simulink model "VCU_CS75_12_30_test"  (R2014a)
settings: Solver=FixedStepDiscrete  StartTime=0.0  StopTime=25  FixedStep=0.0005  RelTol=1e-3
InitFcn:
  | PID_canshu
values from neighbouring files (symbols this model uses):
  D1 = ecucoder_cal(D1)    [PID_canshu.m]
  D2 = ecucoder_cal(D2)    [PID_canshu.m]
  D3 = ecucoder_cal(D3)    [PID_canshu.m]
  ErrorLimit = ecucoder_cal(ErrorLimit)    [PID_canshu.m]
  ErrorSumMax1 = ecucoder_cal(ErrorSumMax1)    [PID_canshu.m]
  ErrorSumMax2 = ecucoder_cal(ErrorSumMax2)    [PID_canshu.m]
  ErrorSumMax3 = ecucoder_cal(ErrorSumMax3)    [PID_canshu.m]
  I1 = ecucoder_cal(I1)    [PID_canshu.m]
  I2 = ecucoder_cal(I2)    [PID_canshu.m]
  I3 = ecucoder_cal(I3)    [PID_canshu.m]
  Limit1 = ecucoder_cal(Limit1)    [PID_canshu.m]
  Limit2 = ecucoder_cal(Limit2)    [PID_canshu.m]
  P1 = ecucoder_cal(P1)    [PID_canshu.m]
  P2 = ecucoder_cal(P2)    [PID_canshu.m]
  P3 = ecucoder_cal(P3)    [PID_canshu.m]
  T_buchang = ecucoder_cal(T_buchang)    [PID_canshu.m]
undefined symbols (not defined in the file or in its folder): ecucoder_acal, I_SW01_L, LaterlAngleCommand, LDW, RemoteAcclPosition
libraries: simulink x940, ec5744lib x41
(part 17 of 31)

== system VCU_CS75_12_30_test/长安CS75底盘程序，20ms一次/Output/CAN1_Tx/to2E5/ACC_2E5/ACC_AEBDecCtrlAvail ==
  ACC_AEBDecCtrlAvail : Inport
  ACC_AEBDecCtrlAvailRon : Rounding  Operator=round
  ACC_AEBDecCtrlAvail_1sat : Saturate  UpperLimit=128  LowerLimit=0
  ACC_AEBDecCtrlAvail_Convert : DataTypeConversion  OutDataTypeStr=uint8
  ACC_AEBDecCtrlAvail_Convert1 : DataTypeConversion  OutDataTypeStr=uint32
  ACC_AEBDecCtrlAvail_D : Product  Inputs=*/
  ACC_AEBDecCtrlAvail_F : Constant  OutDataTypeStr=single
  ACC_AEBDecCtrlAvail_L : simulink/Logic and Bit Operations/Bitwise Operator  logicop=AND  UseBitMask=on  BitMask=128  BitMaskRealWorld=Stored Integer
  ACC_AEBDecCtrlAvail_O : Constant  Value=0  OutDataTypeStr=single
  ACC_AEBDecCtrlAvail_S : ArithShift  BitShiftNumber=-7
  ACC_AEBDecCtrlAvail_sat : Saturate  UpperLimit=1  LowerLimit=0
  ACC_AEBDecCtrlAvail_st : Sum  Inputs=+-
  Constant{1..4,6..8} (7 alike) : Constant  Value=0  OutDataTypeStr=uint8
  output1 : Outport
  output2 : Outport  Port=2
  output3 : Outport  Port=3
  output4 : Outport  Port=4
  output5 : Outport  Port=5
  output6 : Outport  Port=6
  output7 : Outport  Port=7
  output8 : Outport  Port=8
  wires:
  ACC_AEBDecCtrlAvail/1 -> ACC_AEBDecCtrlAvail_sat/1
  ACC_AEBDecCtrlAvail_sat/1 -> ACC_AEBDecCtrlAvail_st/1
  ACC_AEBDecCtrlAvail_O/1 -> ACC_AEBDecCtrlAvail_st/2
  ACC_AEBDecCtrlAvail_st/1 -> ACC_AEBDecCtrlAvail_D/1
  ACC_AEBDecCtrlAvail_F/1 -> ACC_AEBDecCtrlAvail_D/2
  ACC_AEBDecCtrlAvail_D/1 -> ACC_AEBDecCtrlAvailRon/1
  ACC_AEBDecCtrlAvailRon/1 -> ACC_AEBDecCtrlAvail_S/1
  ACC_AEBDecCtrlAvail_S/1 -> ACC_AEBDecCtrlAvail_1sat/1
  ACC_AEBDecCtrlAvail_1sat/1 -> ACC_AEBDecCtrlAvail_Convert1/1
  ACC_AEBDecCtrlAvail_Convert1/1 -> ACC_AEBDecCtrlAvail_L/1
  ACC_AEBDecCtrlAvail_L/1 -> ACC_AEBDecCtrlAvail_Convert/1
  ACC_AEBDecCtrlAvail_Convert/1 -> output5/1
  Constant1/1 -> output1/1
  Constant2/1 -> output2/1
  Constant3/1 -> output3/1
  Constant4/1 -> output4/1
  Constant6/1 -> output6/1
  Constant7/1 -> output7/1
  Constant8/1 -> output8/1

== system VCU_CS75_12_30_test/长安CS75底盘程序，20ms一次/Output/CAN1_Tx/to2E5/ACC_2E5/ACC_AEBLVehilcehold ==
  ACC_AEBLVehilcehold : Inport
  ACC_AEBLVehilceholdRon : Rounding  Operator=round
  ACC_AEBLVehilcehold_1sat : Saturate  UpperLimit=4  LowerLimit=0
  ACC_AEBLVehilcehold_Convert : DataTypeConversion  OutDataTypeStr=uint8
  ACC_AEBLVehilcehold_Convert1 : DataTypeConversion  OutDataTypeStr=uint32
  ACC_AEBLVehilcehold_D : Product  Inputs=*/
  ACC_AEBLVehilcehold_F : Constant  OutDataTypeStr=single
  ACC_AEBLVehilcehold_L : simulink/Logic and Bit Operations/Bitwise Operator  logicop=AND  UseBitMask=on  BitMask=4  BitMaskRealWorld=Stored Integer
  ACC_AEBLVehilcehold_O : Constant  Value=0  OutDataTypeStr=single
  ACC_AEBLVehilcehold_S : ArithShift  BitShiftNumber=-2
  ACC_AEBLVehilcehold_sat : Saturate  UpperLimit=1  LowerLimit=0
  ACC_AEBLVehilcehold_st : Sum  Inputs=+-
  Constant{1..3,5..8} (7 alike) : Constant  Value=0  OutDataTypeStr=uint8
  output1 : Outport
  output2 : Outport  Port=2
  output3 : Outport  Port=3
  output4 : Outport  Port=4
  output5 : Outport  Port=5
  output6 : Outport  Port=6
  output7 : Outport  Port=7
  output8 : Outport  Port=8
  wires:
  ACC_AEBLVehilcehold/1 -> ACC_AEBLVehilcehold_sat/1
  ACC_AEBLVehilcehold_sat/1 -> ACC_AEBLVehilcehold_st/1
  ACC_AEBLVehilcehold_O/1 -> ACC_AEBLVehilcehold_st/2
  ACC_AEBLVehilcehold_st/1 -> ACC_AEBLVehilcehold_D/1
  ACC_AEBLVehilcehold_F/1 -> ACC_AEBLVehilcehold_D/2
  ACC_AEBLVehilcehold_D/1 -> ACC_AEBLVehilceholdRon/1
  ACC_AEBLVehilceholdRon/1 -> ACC_AEBLVehilcehold_S/1
  ACC_AEBLVehilcehold_S/1 -> ACC_AEBLVehilcehold_1sat/1
  ACC_AEBLVehilcehold_1sat/1 -> ACC_AEBLVehilcehold_Convert1/1
  ACC_AEBLVehilcehold_Convert1/1 -> ACC_AEBLVehilcehold_L/1
  ACC_AEBLVehilcehold_L/1 -> ACC_AEBLVehilcehold_Convert/1
  ACC_AEBLVehilcehold_Convert/1 -> output4/1
  Constant1/1 -> output1/1
  Constant2/1 -> output2/1
  Constant3/1 -> output3/1
  Constant5/1 -> output5/1
  Constant6/1 -> output6/1
  Constant7/1 -> output7/1
  Constant8/1 -> output8/1

== system VCU_CS75_12_30_test/长安CS75底盘程序，20ms一次/Output/CAN1_Tx/to2E5/ACC_2E5/ACC_AEBTargetDeceleration ==
  ACC_AEBTargetDeceleration : Inport
  ACC_AEBTargetDecelerationBitCov : DataTypeConversion  OutDataTypeStr=uint32
  ACC_AEBTargetDecelerationBitCov1 : DataTypeConversion  OutDataTypeStr=uint8
  ACC_AEBTargetDecelerationCOV : DataTypeConversion  OutDataTypeStr=uint8
  ACC_AEBTargetDecelerationCOV1 : DataTypeConversion  OutDataTypeStr=uint8
  ACC_AEBTargetDecelerationRon : Rounding  Operator=round
  ACC_AEBTargetDeceleration_1sat : Saturate  UpperLimit=2097120  LowerLimit=0
  ACC_AEBTargetDeceleration_And : simulink/Logic and Bit Operations/Bitwise Operator  logicop=AND  UseBitMask=off  NumInputPorts=2  BitMask=bin2dec('11011001')  BitMaskRealWorld=Stored Integer
  ACC_AEBTargetDeceleration_And1 : simulink/Logic and Bit Operations/Bitwise Operator  logicop=AND  UseBitMask=off  NumInputPorts=2  BitMask=bin2dec('11011001')  BitMaskRealWorld=Stored Integer
  ACC_AEBTargetDeceleration_And1_C : Constant  Value=255  OutDataTypeStr=uint32
  ACC_AEBTargetDeceleration_And_C : Constant  Value=65535
  ACC_AEBTargetDeceleration_Convert : DataTypeConversion  OutDataTypeStr=uint32
  ACC_AEBTargetDeceleration_D : Product  Inputs=*/
  ACC_AEBTargetDeceleration_D1 : Product  Inputs=*/
  ACC_AEBTargetDeceleration_D2 : Product  Inputs=*/
  ACC_AEBTargetDeceleration_F : Constant  Value=0.0005  OutDataTypeStr=single
  ACC_AEBTargetDeceleration_L : simulink/Logic and Bit Operations/Bitwise Operator  logicop=AND  UseBitMask=on  BitMask=2097120  BitMaskRealWorld=Stored Integer
  ACC_AEBTargetDeceleration_O : Constant  Value=-16  OutDataTypeStr=single
  ACC_AEBTargetDeceleration_S : ArithShift  BitShiftNumber=-5
  ACC_AEBTargetDeceleration_sat : Saturate  UpperLimit=16  LowerLimit=-16
  ACC_AEBTargetDeceleration_st : Sum  Inputs=+-
  ACC_AEBTargetDecelerationoutput1_C : Constant  Value=65536
  ACC_AEBTargetDecelerationoutput2_C : Constant  Value=256
  Constant{4..8} (5 alike) : Constant  Value=0  OutDataTypeStr=uint8
  output1 : Outport
  output2 : Outport  Port=2
  output3 : Outport  Port=3
  output4 : Outport  Port=4
  output5 : Outport  Port=5
  output6 : Outport  Port=6
  output7 : Outport  Port=7
  output8 : Outport  Port=8
  wires:
  ACC_AEBTargetDeceleration/1 -> ACC_AEBTargetDeceleration_sat/1
  ACC_AEBTargetDeceleration_sat/1 -> ACC_AEBTargetDeceleration_st/1
  ACC_AEBTargetDeceleration_O/1 -> ACC_AEBTargetDeceleration_st/2
  ACC_AEBTargetDeceleration_st/1 -> ACC_AEBTargetDeceleration_D/1
  ACC_AEBTargetDeceleration_F/1 -> ACC_AEBTargetDeceleration_D/2
  ACC_AEBTargetDeceleration_D/1 -> ACC_AEBTargetDecelerationRon/1
  ACC_AEBTargetDecelerationRon/1 -> ACC_AEBTargetDeceleration_S/1
  ACC_AEBTargetDeceleration_S/1 -> ACC_AEBTargetDeceleration_1sat/1
  ACC_AEBTargetDeceleration_1sat/1 -> ACC_AEBTargetDeceleration_Convert/1
  ACC_AEBTargetDeceleration_Convert/1 -> ACC_AEBTargetDeceleration_L/1
  ACC_AEBTargetDeceleration_L/1 -> ACC_AEBTargetDeceleration_D1/1, ACC_AEBTargetDeceleration_And/1, ACC_AEBTargetDeceleration_And1/1
  ACC_AEBTargetDecelerationoutput1_C/1 -> ACC_AEBTargetDeceleration_D1/2
  ACC_AEBTargetDeceleration_D1/1 -> ACC_AEBTargetDecelerationCOV/1
  ACC_AEBTargetDecelerationCOV/1 -> output1/1
  ACC_AEBTargetDeceleration_And_C/1 -> ACC_AEBTargetDecelerationBitCov/1
  ACC_AEBTargetDecelerationBitCov/1 -> ACC_AEBTargetDeceleration_And/2
  ACC_AEBTargetDeceleration_And/1 -> ACC_AEBTargetDeceleration_D2/1
  ACC_AEBTargetDecelerationoutput2_C/1 -> ACC_AEBTargetDeceleration_D2/2
  ACC_AEBTargetDeceleration_D2/1 -> ACC_AEBTargetDecelerationCOV1/1
  ACC_AEBTargetDecelerationCOV1/1 -> output2/1
  ACC_AEBTargetDeceleration_And1_C/1 -> ACC_AEBTargetDeceleration_And1/2
  ACC_AEBTargetDeceleration_And1/1 -> ACC_AEBTargetDecelerationBitCov1/1
  ACC_AEBTargetDecelerationBitCov1/1 -> output3/1
  Constant4/1 -> output4/1
  Constant5/1 -> output5/1
  Constant6/1 -> output6/1
  Constant7/1 -> output7/1
  Constant8/1 -> output8/1

== system VCU_CS75_12_30_test/长安CS75底盘程序，20ms一次/Output/CAN1_Tx/to2E5/ACC_2E5/ACC_AWBavailable ==
  ACC_AWBavailable : Inport
  ACC_AWBavailableRon : Rounding  Operator=round
  ACC_AWBavailable_1sat : Saturate  UpperLimit=128  LowerLimit=0
  ACC_AWBavailable_Convert : DataTypeConversion  OutDataTypeStr=uint8
  ACC_AWBavailable_Convert1 : DataTypeConversion  OutDataTypeStr=uint32
  ACC_AWBavailable_D : Product  Inputs=*/
  ACC_AWBavailable_F : Constant  OutDataTypeStr=single
  ACC_AWBavailable_L : simulink/Logic and Bit Operations/Bitwise Operator  logicop=AND  UseBitMask=on  BitMask=128  BitMaskRealWorld=Stored Integer
  ACC_AWBavailable_O : Constant  Value=0  OutDataTypeStr=single
  ACC_AWBavailable_S : ArithShift  BitShiftNumber=-7
  ACC_AWBavailable_sat : Saturate  UpperLimit=1  LowerLimit=0
  ACC_AWBavailable_st : Sum  Inputs=+-
  Constant{1..3,5..8} (7 alike) : Constant  Value=0  OutDataTypeStr=uint8
  output1 : Outport
  output2 : Outport  Port=2
  output3 : Outport  Port=3
  output4 : Outport  Port=4
  output5 : Outport  Port=5
  output6 : Outport  Port=6
  output7 : Outport  Port=7
  output8 : Outport  Port=8
  wires:
  ACC_AWBavailable/1 -> ACC_AWBavailable_sat/1
  ACC_AWBavailable_sat/1 -> ACC_AWBavailable_st/1
  ACC_AWBavailable_O/1 -> ACC_AWBavailable_st/2
  ACC_AWBavailable_st/1 -> ACC_AWBavailable_D/1
  ACC_AWBavailable_F/1 -> ACC_AWBavailable_D/2
  ACC_AWBavailable_D/1 -> ACC_AWBavailableRon/1
  ACC_AWBavailableRon/1 -> ACC_AWBavailable_S/1
  ACC_AWBavailable_S/1 -> ACC_AWBavailable_1sat/1
  ACC_AWBavailable_1sat/1 -> ACC_AWBavailable_Convert1/1
  ACC_AWBavailable_Convert1/1 -> ACC_AWBavailable_L/1
  ACC_AWBavailable_L/1 -> ACC_AWBavailable_Convert/1
  ACC_AWBavailable_Convert/1 -> output4/1
  Constant1/1 -> output1/1
  Constant2/1 -> output2/1
  Constant3/1 -> output3/1
  Constant5/1 -> output5/1
  Constant6/1 -> output6/1
  Constant7/1 -> output7/1
  Constant8/1 -> output8/1

== system VCU_CS75_12_30_test/长安CS75底盘程序，20ms一次/Output/CAN1_Tx/to2E5/ACC_2E5/ACC_AWBlevel ==
  ACC_AWBlevel : Inport
  ACC_AWBlevelRon : Rounding  Operator=round
  ACC_AWBlevel_1sat : Saturate  UpperLimit=15  LowerLimit=0
  ACC_AWBlevel_Convert : DataTypeConversion  OutDataTypeStr=uint8
  ACC_AWBlevel_Convert1 : DataTypeConversion  OutDataTypeStr=uint32
  ACC_AWBlevel_D : Product  Inputs=*/
  ACC_AWBlevel_F : Constant  OutDataTypeStr=single
  ACC_AWBlevel_L : simulink/Logic and Bit Operations/Bitwise Operator  logicop=AND  UseBitMask=on  BitMask=15  BitMaskRealWorld=Stored Integer
  ACC_AWBlevel_O : Constant  Value=0  OutDataTypeStr=single
  ACC_AWBlevel_S : ArithShift
  ACC_AWBlevel_sat : Saturate  UpperLimit=15  LowerLimit=0
  ACC_AWBlevel_st : Sum  Inputs=+-
  Constant{1..2,4..8} (7 alike) : Constant  Value=0  OutDataTypeStr=uint8
  output1 : Outport
  output2 : Outport  Port=2
  output3 : Outport  Port=3
  output4 : Outport  Port=4
  output5 : Outport  Port=5
  output6 : Outport  Port=6
  output7 : Outport  Port=7
  output8 : Outport  Port=8
  wires:
  ACC_AWBlevel/1 -> ACC_AWBlevel_sat/1
  ACC_AWBlevel_sat/1 -> ACC_AWBlevel_st/1
  ACC_AWBlevel_O/1 -> ACC_AWBlevel_st/2
  ACC_AWBlevel_st/1 -> ACC_AWBlevel_D/1
  ACC_AWBlevel_F/1 -> ACC_AWBlevel_D/2
  ACC_AWBlevel_D/1 -> ACC_AWBlevelRon/1
  ACC_AWBlevelRon/1 -> ACC_AWBlevel_S/1
  ACC_AWBlevel_S/1 -> ACC_AWBlevel_1sat/1
  ACC_AWBlevel_1sat/1 -> ACC_AWBlevel_Convert1/1
  ACC_AWBlevel_Convert1/1 -> ACC_AWBlevel_L/1
  ACC_AWBlevel_L/1 -> ACC_AWBlevel_Convert/1
  ACC_AWBlevel_Convert/1 -> output3/1
  Constant1/1 -> output1/1
  Constant2/1 -> output2/1
  Constant4/1 -> output4/1
  Constant5/1 -> output5/1
  Constant6/1 -> output6/1
  Constant7/1 -> output7/1
  Constant8/1 -> output8/1

== system VCU_CS75_12_30_test/长安CS75底盘程序，20ms一次/Output/CAN1_Tx/to2E5/ACC_2E5/ACC_AccTorqueReq ==
  ACC_AccTorqueReq : Inport
  ACC_AccTorqueReqBitCov : DataTypeConversion  OutDataTypeStr=uint8
  ACC_AccTorqueReqCOV : DataTypeConversion  OutDataTypeStr=uint8
  ACC_AccTorqueReqRon : Rounding  Operator=round
  ACC_AccTorqueReq_1sat : Saturate  UpperLimit=4092  LowerLimit=0
  ACC_AccTorqueReq_And : simulink/Logic and Bit Operations/Bitwise Operator  logicop=AND  UseBitMask=off  NumInputPorts=2  BitMask=bin2dec('11011001')  BitMaskRealWorld=Stored Integer
  ACC_AccTorqueReq_And_C : Constant  Value=255  OutDataTypeStr=uint32
  ACC_AccTorqueReq_Convert : DataTypeConversion  OutDataTypeStr=uint32
  ACC_AccTorqueReq_D : Product  Inputs=*/
  ACC_AccTorqueReq_D1 : Product  Inputs=*/
  ACC_AccTorqueReq_F : Constant  Value=0.09784  OutDataTypeStr=single
  ACC_AccTorqueReq_L : simulink/Logic and Bit Operations/Bitwise Operator  logicop=AND  UseBitMask=on  BitMask=4092  BitMaskRealWorld=Stored Integer
  ACC_AccTorqueReq_O : Constant  Value=0  OutDataTypeStr=single
  ACC_AccTorqueReq_S : ArithShift  BitShiftNumber=-2
  ACC_AccTorqueReq_sat : Saturate  UpperLimit=100.09032  LowerLimit=0
  ACC_AccTorqueReq_st : Sum  Inputs=+-
  ACC_AccTorqueReqoutput5_C : Constant  Value=256
  Constant{1..4,7..8} (6 alike) : Constant  Value=0  OutDataTypeStr=uint8
  output1 : Outport
  output2 : Outport  Port=2
  output3 : Outport  Port=3
  output4 : Outport  Port=4
  output5 : Outport  Port=5
  output6 : Outport  Port=6
  output7 : Outport  Port=7
  output8 : Outport  Port=8
  wires:
  ACC_AccTorqueReq/1 -> ACC_AccTorqueReq_sat/1
  ACC_AccTorqueReq_sat/1 -> ACC_AccTorqueReq_st/1
  ACC_AccTorqueReq_O/1 -> ACC_AccTorqueReq_st/2
  ACC_AccTorqueReq_st/1 -> ACC_AccTorqueReq_D/1
  ACC_AccTorqueReq_F/1 -> ACC_AccTorqueReq_D/2
  ACC_AccTorqueReq_D/1 -> ACC_AccTorqueReqRon/1
  ACC_AccTorqueReqRon/1 -> ACC_AccTorqueReq_S/1
  ACC_AccTorqueReq_S/1 -> ACC_AccTorqueReq_1sat/1
  ACC_AccTorqueReq_1sat/1 -> ACC_AccTorqueReq_Convert/1
  ACC_AccTorqueReq_Convert/1 -> ACC_AccTorqueReq_L/1
  ACC_AccTorqueReq_L/1 -> ACC_AccTorqueReq_D1/1, ACC_AccTorqueReq_And/1
  ACC_AccTorqueReqoutput5_C/1 -> ACC_AccTorqueReq_D1/2
  ACC_AccTorqueReq_D1/1 -> ACC_AccTorqueReqCOV/1
  ACC_AccTorqueReqCOV/1 -> output5/1
  ACC_AccTorqueReq_And_C/1 -> ACC_AccTorqueReq_And/2
  ACC_AccTorqueReq_And/1 -> ACC_AccTorqueReqBitCov/1
  ACC_AccTorqueReqBitCov/1 -> output6/1
  Constant1/1 -> output1/1
  Constant2/1 -> output2/1
  Constant3/1 -> output3/1
  Constant4/1 -> output4/1
  Constant7/1 -> output7/1
  Constant8/1 -> output8/1

== system VCU_CS75_12_30_test/长安CS75底盘程序，20ms一次/Output/CAN1_Tx/to2E5/ACC_2E5/ACC_AccTrqReqEnable ==
  ACC_AccTrqReqEnable : Inport
  ACC_AccTrqReqEnableRon : Rounding  Operator=round
  ACC_AccTrqReqEnable_1sat : Saturate  UpperLimit=128  LowerLimit=0
  ACC_AccTrqReqEnable_Convert : DataTypeConversion  OutDataTypeStr=uint8
  ACC_AccTrqReqEnable_Convert1 : DataTypeConversion  OutDataTypeStr=uint32
  ACC_AccTrqReqEnable_D : Product  Inputs=*/
  ACC_AccTrqReqEnable_F : Constant  OutDataTypeStr=single
  ACC_AccTrqReqEnable_L : simulink/Logic and Bit Operations/Bitwise Operator  logicop=AND  UseBitMask=on  BitMask=128  BitMaskRealWorld=Stored Integer
  ACC_AccTrqReqEnable_O : Constant  Value=0  OutDataTypeStr=single
  ACC_AccTrqReqEnable_S : ArithShift  BitShiftNumber=-7
  ACC_AccTrqReqEnable_sat : Saturate  UpperLimit=1  LowerLimit=0
  ACC_AccTrqReqEnable_st : Sum  Inputs=+-
  Constant{2..8} (7 alike) : Constant  Value=0  OutDataTypeStr=uint8
  output1 : Outport
  output2 : Outport  Port=2
  output3 : Outport  Port=3
  output4 : Outport  Port=4
  output5 : Outport  Port=5
  output6 : Outport  Port=6
  output7 : Outport  Port=7
  output8 : Outport  Port=8
  wires:
  ACC_AccTrqReqEnable/1 -> ACC_AccTrqReqEnable_sat/1
  ACC_AccTrqReqEnable_sat/1 -> ACC_AccTrqReqEnable_st/1
  ACC_AccTrqReqEnable_O/1 -> ACC_AccTrqReqEnable_st/2
  ACC_AccTrqReqEnable_st/1 -> ACC_AccTrqReqEnable_D/1
  ACC_AccTrqReqEnable_F/1 -> ACC_AccTrqReqEnable_D/2
  ACC_AccTrqReqEnable_D/1 -> ACC_AccTrqReqEnableRon/1
  ACC_AccTrqReqEnableRon/1 -> ACC_AccTrqReqEnable_S/1
  ACC_AccTrqReqEnable_S/1 -> ACC_AccTrqReqEnable_1sat/1
  ACC_AccTrqReqEnable_1sat/1 -> ACC_AccTrqReqEnable_Convert1/1
  ACC_AccTrqReqEnable_Convert1/1 -> ACC_AccTrqReqEnable_L/1
  ACC_AccTrqReqEnable_L/1 -> ACC_AccTrqReqEnable_Convert/1
  ACC_AccTrqReqEnable_Convert/1 -> output1/1
  Constant2/1 -> output2/1
  Constant3/1 -> output3/1
  Constant4/1 -> output4/1
  Constant5/1 -> output5/1
  Constant6/1 -> output6/1
  Constant7/1 -> output7/1
  Constant8/1 -> output8/1

== system VCU_CS75_12_30_test/长安CS75底盘程序，20ms一次/Output/CAN1_Tx/to2E5/ACC_2E5/ACC_CheckSum ==
  ACC_CheckSum : Inport
  ACC_CheckSumRon : Rounding  Operator=round
  ACC_CheckSum_1sat : Saturate  UpperLimit=255  LowerLimit=0
  ACC_CheckSum_Convert : DataTypeConversion  OutDataTypeStr=uint8
  ACC_CheckSum_Convert1 : DataTypeConversion  OutDataTypeStr=uint32
  ACC_CheckSum_D : Product  Inputs=*/
  ACC_CheckSum_F : Constant  OutDataTypeStr=single
  ACC_CheckSum_L : simulink/Logic and Bit Operations/Bitwise Operator  logicop=AND  UseBitMask=on  BitMask=255  BitMaskRealWorld=Stored Integer
  ACC_CheckSum_O : Constant  Value=0  OutDataTypeStr=single
  ACC_CheckSum_S : ArithShift
  ACC_CheckSum_sat : Saturate  UpperLimit=255  LowerLimit=0
  ACC_CheckSum_st : Sum  Inputs=+-
  Constant{1..7} (7 alike) : Constant  Value=0  OutDataTypeStr=uint8
  output1 : Outport
  output2 : Outport  Port=2
  output3 : Outport  Port=3
  output4 : Outport  Port=4
  output5 : Outport  Port=5
  output6 : Outport  Port=6
  output7 : Outport  Port=7
  output8 : Outport  Port=8
  wires:
  ACC_CheckSum/1 -> ACC_CheckSum_sat/1
  ACC_CheckSum_sat/1 -> ACC_CheckSum_st/1
  ACC_CheckSum_O/1 -> ACC_CheckSum_st/2
  ACC_CheckSum_st/1 -> ACC_CheckSum_D/1
  ACC_CheckSum_F/1 -> ACC_CheckSum_D/2
  ACC_CheckSum_D/1 -> ACC_CheckSumRon/1
  ACC_CheckSumRon/1 -> ACC_CheckSum_S/1
  ACC_CheckSum_S/1 -> ACC_CheckSum_1sat/1
  ACC_CheckSum_1sat/1 -> ACC_CheckSum_Convert1/1
  ACC_CheckSum_Convert1/1 -> ACC_CheckSum_L/1
  ACC_CheckSum_L/1 -> ACC_CheckSum_Convert/1
  ACC_CheckSum_Convert/1 -> output8/1
  Constant1/1 -> output1/1
  Constant2/1 -> output2/1
  Constant3/1 -> output3/1
  Constant4/1 -> output4/1
  Constant5/1 -> output5/1
  Constant6/1 -> output6/1
  Constant7/1 -> output7/1

== system VCU_CS75_12_30_test/长安CS75底盘程序，20ms一次/Output/CAN1_Tx/to2E5/ACC_2E5/ACC_ESPPrefill ==
  ACC_ESPPrefill : Inport
  ACC_ESPPrefillRon : Rounding  Operator=round
  ACC_ESPPrefill_1sat : Saturate  UpperLimit=64  LowerLimit=0
  ACC_ESPPrefill_Convert : DataTypeConversion  OutDataTypeStr=uint8
  ACC_ESPPrefill_Convert1 : DataTypeConversion  OutDataTypeStr=uint32
  ACC_ESPPrefill_D : Product  Inputs=*/
  ACC_ESPPrefill_F : Constant  OutDataTypeStr=single
  ACC_ESPPrefill_L : simulink/Logic and Bit Operations/Bitwise Operator  logicop=AND  UseBitMask=on  BitMask=64  BitMaskRealWorld=Stored Integer
  ACC_ESPPrefill_O : Constant  Value=0  OutDataTypeStr=single
  ACC_ESPPrefill_S : ArithShift  BitShiftNumber=-6
  ACC_ESPPrefill_sat : Saturate  UpperLimit=1  LowerLimit=0
  ACC_ESPPrefill_st : Sum  Inputs=+-
  Constant{1..3,5..8} (7 alike) : Constant  Value=0  OutDataTypeStr=uint8
  output1 : Outport
  output2 : Outport  Port=2
  output3 : Outport  Port=3
  output4 : Outport  Port=4
  output5 : Outport  Port=5
  output6 : Outport  Port=6
  output7 : Outport  Port=7
  output8 : Outport  Port=8
  wires:
  ACC_ESPPrefill/1 -> ACC_ESPPrefill_sat/1
  ACC_ESPPrefill_sat/1 -> ACC_ESPPrefill_st/1
  ACC_ESPPrefill_O/1 -> ACC_ESPPrefill_st/2
  ACC_ESPPrefill_st/1 -> ACC_ESPPrefill_D/1
  ACC_ESPPrefill_F/1 -> ACC_ESPPrefill_D/2
  ACC_ESPPrefill_D/1 -> ACC_ESPPrefillRon/1
  ACC_ESPPrefillRon/1 -> ACC_ESPPrefill_S/1
  ACC_ESPPrefill_S/1 -> ACC_ESPPrefill_1sat/1
  ACC_ESPPrefill_1sat/1 -> ACC_ESPPrefill_Convert1/1
  ACC_ESPPrefill_Convert1/1 -> ACC_ESPPrefill_L/1
  ACC_ESPPrefill_L/1 -> ACC_ESPPrefill_Convert/1
  ACC_ESPPrefill_Convert/1 -> output4/1
  Constant1/1 -> output1/1
  Constant2/1 -> output2/1
  Constant3/1 -> output3/1
  Constant5/1 -> output5/1
  Constant6/1 -> output6/1
  Constant7/1 -> output7/1
  Constant8/1 -> output8/1

== system VCU_CS75_12_30_test/长安CS75底盘程序，20ms一次/Output/CAN1_Tx/to2E5/ACC_2E5/ACC_PCWPenable ==
  ACC_PCWPenable : Inport
  ACC_PCWPenableRon : Rounding  Operator=round
  ACC_PCWPenable_1sat : Saturate  UpperLimit=32  LowerLimit=0
  ACC_PCWPenable_Convert : DataTypeConversion  OutDataTypeStr=uint8
  ACC_PCWPenable_Convert1 : DataTypeConversion  OutDataTypeStr=uint32
  ACC_PCWPenable_D : Product  Inputs=*/
  ACC_PCWPenable_F : Constant  OutDataTypeStr=single
  ACC_PCWPenable_L : simulink/Logic and Bit Operations/Bitwise Operator  logicop=AND  UseBitMask=on  BitMask=32  BitMaskRealWorld=Stored Integer
  ACC_PCWPenable_O : Constant  Value=0  OutDataTypeStr=single
  ACC_PCWPenable_S : ArithShift  BitShiftNumber=-5
  ACC_PCWPenable_sat : Saturate  UpperLimit=1  LowerLimit=0
  ACC_PCWPenable_st : Sum  Inputs=+-
  Constant{1..3,5..8} (7 alike) : Constant  Value=0  OutDataTypeStr=uint8
  output1 : Outport
  output2 : Outport  Port=2
  output3 : Outport  Port=3
  output4 : Outport  Port=4
  output5 : Outport  Port=5
  output6 : Outport  Port=6
  output7 : Outport  Port=7
  output8 : Outport  Port=8
  wires:
  ACC_PCWPenable/1 -> ACC_PCWPenable_sat/1
  ACC_PCWPenable_sat/1 -> ACC_PCWPenable_st/1
  ACC_PCWPenable_O/1 -> ACC_PCWPenable_st/2
  ACC_PCWPenable_st/1 -> ACC_PCWPenable_D/1
  ACC_PCWPenable_F/1 -> ACC_PCWPenable_D/2
  ACC_PCWPenable_D/1 -> ACC_PCWPenableRon/1
  ACC_PCWPenableRon/1 -> ACC_PCWPenable_S/1
  ACC_PCWPenable_S/1 -> ACC_PCWPenable_1sat/1
  ACC_PCWPenable_1sat/1 -> ACC_PCWPenable_Convert1/1
  ACC_PCWPenable_Convert1/1 -> ACC_PCWPenable_L/1
  ACC_PCWPenable_L/1 -> ACC_PCWPenable_Convert/1
  ACC_PCWPenable_Convert/1 -> output4/1
  Constant1/1 -> output1/1
  Constant2/1 -> output2/1
  Constant3/1 -> output3/1
  Constant5/1 -> output5/1
  Constant6/1 -> output6/1
  Constant7/1 -> output7/1
  Constant8/1 -> output8/1

== system VCU_CS75_12_30_test/长安CS75底盘程序，20ms一次/Output/CAN1_Tx/to2E5/ACC_2E5/ACC_PCWPreWarning ==
  ACC_PCWPreWarning : Inport
  ACC_PCWPreWarningRon : Rounding  Operator=round
  ACC_PCWPreWarning_1sat : Saturate  UpperLimit=8  LowerLimit=0
  ACC_PCWPreWarning_Convert : DataTypeConversion  OutDataTypeStr=uint8
  ACC_PCWPreWarning_Convert1 : DataTypeConversion  OutDataTypeStr=uint32
  ACC_PCWPreWarning_D : Product  Inputs=*/
  ACC_PCWPreWarning_F : Constant  OutDataTypeStr=single
  ACC_PCWPreWarning_L : simulink/Logic and Bit Operations/Bitwise Operator  logicop=AND  UseBitMask=on  BitMask=8  BitMaskRealWorld=Stored Integer
  ACC_PCWPreWarning_O : Constant  Value=0  OutDataTypeStr=single
  ACC_PCWPreWarning_S : ArithShift  BitShiftNumber=-3
  ACC_PCWPreWarning_sat : Saturate  UpperLimit=0  LowerLimit=0
  ACC_PCWPreWarning_st : Sum  Inputs=+-
  Constant{1..3,5..8} (7 alike) : Constant  Value=0  OutDataTypeStr=uint8
  output1 : Outport
  output2 : Outport  Port=2
  output3 : Outport  Port=3
  output4 : Outport  Port=4
  output5 : Outport  Port=5
  output6 : Outport  Port=6
  output7 : Outport  Port=7
  output8 : Outport  Port=8
  wires:
  ACC_PCWPreWarning/1 -> ACC_PCWPreWarning_sat/1
  ACC_PCWPreWarning_sat/1 -> ACC_PCWPreWarning_st/1
  ACC_PCWPreWarning_O/1 -> ACC_PCWPreWarning_st/2
  ACC_PCWPreWarning_st/1 -> ACC_PCWPreWarning_D/1
  ACC_PCWPreWarning_F/1 -> ACC_PCWPreWarning_D/2
  ACC_PCWPreWarning_D/1 -> ACC_PCWPreWarningRon/1
  ACC_PCWPreWarningRon/1 -> ACC_PCWPreWarning_S/1
  ACC_PCWPreWarning_S/1 -> ACC_PCWPreWarning_1sat/1
  ACC_PCWPreWarning_1sat/1 -> ACC_PCWPreWarning_Convert1/1
  ACC_PCWPreWarning_Convert1/1 -> ACC_PCWPreWarning_L/1
  ACC_PCWPreWarning_L/1 -> ACC_PCWPreWarning_Convert/1
  ACC_PCWPreWarning_Convert/1 -> output4/1
  Constant1/1 -> output1/1
  Constant2/1 -> output2/1
  Constant3/1 -> output3/1
  Constant5/1 -> output5/1
  Constant6/1 -> output6/1
  Constant7/1 -> output7/1
  Constant8/1 -> output8/1

== system VCU_CS75_12_30_test/长安CS75底盘程序，20ms一次/Output/CAN1_Tx/to2E5/ACC_2E5/ACC_PCW_LatentWarning ==
  ACC_PCW_LatentWarning : Inport
  ACC_PCW_LatentWarningRon : Rounding  Operator=round
  ACC_PCW_LatentWarning_1sat : Saturate  UpperLimit=16  LowerLimit=0
  ACC_PCW_LatentWarning_Convert : DataTypeConversion  OutDataTypeStr=uint8
  ACC_PCW_LatentWarning_Convert1 : DataTypeConversion  OutDataTypeStr=uint32
  ACC_PCW_LatentWarning_D : Product  Inputs=*/
  ACC_PCW_LatentWarning_F : Constant  OutDataTypeStr=single
  ACC_PCW_LatentWarning_L : simulink/Logic and Bit Operations/Bitwise Operator  logicop=AND  UseBitMask=on  BitMask=16  BitMaskRealWorld=Stored Integer
  ACC_PCW_LatentWarning_O : Constant  Value=0  OutDataTypeStr=single
  ACC_PCW_LatentWarning_S : ArithShift  BitShiftNumber=-4
  ACC_PCW_LatentWarning_sat : Saturate  UpperLimit=0  LowerLimit=0
  ACC_PCW_LatentWarning_st : Sum  Inputs=+-
  Constant{1..3,5..8} (7 alike) : Constant  Value=0  OutDataTypeStr=uint8
  output1 : Outport
  output2 : Outport  Port=2
  output3 : Outport  Port=3
  output4 : Outport  Port=4
  output5 : Outport  Port=5
  output6 : Outport  Port=6
  output7 : Outport  Port=7
  output8 : Outport  Port=8
  wires:
  ACC_PCW_LatentWarning/1 -> ACC_PCW_LatentWarning_sat/1
  ACC_PCW_LatentWarning_sat/1 -> ACC_PCW_LatentWarning_st/1
  ACC_PCW_LatentWarning_O/1 -> ACC_PCW_LatentWarning_st/2
  ACC_PCW_LatentWarning_st/1 -> ACC_PCW_LatentWarning_D/1
  ACC_PCW_LatentWarning_F/1 -> ACC_PCW_LatentWarning_D/2
  ACC_PCW_LatentWarning_D/1 -> ACC_PCW_LatentWarningRon/1
  ACC_PCW_LatentWarningRon/1 -> ACC_PCW_LatentWarning_S/1
  ACC_PCW_LatentWarning_S/1 -> ACC_PCW_LatentWarning_1sat/1
  ACC_PCW_LatentWarning_1sat/1 -> ACC_PCW_LatentWarning_Convert1/1
  ACC_PCW_LatentWarning_Convert1/1 -> ACC_PCW_LatentWarning_L/1
  ACC_PCW_LatentWarning_L/1 -> ACC_PCW_LatentWarning_Convert/1
  ACC_PCW_LatentWarning_Convert/1 -> output4/1
  Constant1/1 -> output1/1
  Constant2/1 -> output2/1
  Constant3/1 -> output3/1
  Constant5/1 -> output5/1
  Constant6/1 -> output6/1
  Constant7/1 -> output7/1
  Constant8/1 -> output8/1

== system VCU_CS75_12_30_test/长安CS75底盘程序，20ms一次/Output/CAN1_Tx/to2E5/ACC_2E5/ACC_RollingCounter ==
  ACC_RollingCounter : Inport
  ACC_RollingCounterRon : Rounding  Operator=round
  ACC_RollingCounter_1sat : Saturate  UpperLimit=15  LowerLimit=0
  ACC_RollingCounter_Convert : DataTypeConversion  OutDataTypeStr=uint8
  ACC_RollingCounter_Convert1 : DataTypeConversion  OutDataTypeStr=uint32
  ACC_RollingCounter_D : Product  Inputs=*/
  ACC_RollingCounter_F : Constant  OutDataTypeStr=single
  ACC_RollingCounter_L : simulink/Logic and Bit Operations/Bitwise Operator  logicop=AND  UseBitMask=on  BitMask=15  BitMaskRealWorld=Stored Integer
  ACC_RollingCounter_O : Constant  Value=0  OutDataTypeStr=single
  ACC_RollingCounter_S : ArithShift
  ACC_RollingCounter_sat : Saturate  UpperLimit=15  LowerLimit=0
  ACC_RollingCounter_st : Sum  Inputs=+-
  Constant{1..6,8} (7 alike) : Constant  Value=0  OutDataTypeStr=uint8
  output1 : Outport
  output2 : Outport  Port=2
  output3 : Outport  Port=3
  output4 : Outport  Port=4
  output5 : Outport  Port=5
  output6 : Outport  Port=6
  output7 : Outport  Port=7
  output8 : Outport  Port=8
  wires:
  ACC_RollingCounter/1 -> ACC_RollingCounter_sat/1
  ACC_RollingCounter_sat/1 -> ACC_RollingCounter_st/1
  ACC_RollingCounter_O/1 -> ACC_RollingCounter_st/2
  ACC_RollingCounter_st/1 -> ACC_RollingCounter_D/1
  ACC_RollingCounter_F/1 -> ACC_RollingCounter_D/2
  ACC_RollingCounter_D/1 -> ACC_RollingCounterRon/1
  ACC_RollingCounterRon/1 -> ACC_RollingCounter_S/1
  ACC_RollingCounter_S/1 -> ACC_RollingCounter_1sat/1
  ACC_RollingCounter_1sat/1 -> ACC_RollingCounter_Convert1/1
  ACC_RollingCounter_Convert1/1 -> ACC_RollingCounter_L/1
  ACC_RollingCounter_L/1 -> ACC_RollingCounter_Convert/1
  ACC_RollingCounter_Convert/1 -> output7/1
  Constant1/1 -> output1/1
  Constant2/1 -> output2/1
  Constant3/1 -> output3/1
  Constant4/1 -> output4/1
  Constant5/1 -> output5/1
  Constant6/1 -> output6/1
  Constant8/1 -> output8/1

== system VCU_CS75_12_30_test/长安CS75底盘程序，20ms一次/Output/CAN1_Tx/to2E5/ACC_2E5/ACC_TextInfoForDriver ==
  ACC_TextInfoForDriver : Inport
  ACC_TextInfoForDriverBitCov : DataTypeConversion  OutDataTypeStr=uint8
  ACC_TextInfoForDriverCOV : DataTypeConversion  OutDataTypeStr=uint8
  ACC_TextInfoForDriverRon : Rounding  Operator=round
  ACC_TextInfoForDriver_1sat : Saturate  UpperLimit=992  LowerLimit=0
  ACC_TextInfoForDriver_And : simulink/Logic and Bit Operations/Bitwise Operator  logicop=AND  UseBitMask=off  NumInputPorts=2  BitMask=bin2dec('11011001')  BitMaskRealWorld=Stored Integer
  ACC_TextInfoForDriver_And_C : Constant  Value=255  OutDataTypeStr=uint32
  ACC_TextInfoForDriver_Convert : DataTypeConversion  OutDataTypeStr=uint32
  ACC_TextInfoForDriver_D : Product  Inputs=*/
  ACC_TextInfoForDriver_D1 : Product  Inputs=*/
  ACC_TextInfoForDriver_F : Constant  OutDataTypeStr=single
  ACC_TextInfoForDriver_L : simulink/Logic and Bit Operations/Bitwise Operator  logicop=AND  UseBitMask=on  BitMask=992  BitMaskRealWorld=Stored Integer
  ACC_TextInfoForDriver_O : Constant  Value=0  OutDataTypeStr=single
  ACC_TextInfoForDriver_S : ArithShift  BitShiftNumber=-5
  ACC_TextInfoForDriver_sat : Saturate  UpperLimit=31  LowerLimit=0
  ACC_TextInfoForDriver_st : Sum  Inputs=+-
  ACC_TextInfoForDriveroutput6_C : Constant  Value=256
  Constant{1..5,8} (6 alike) : Constant  Value=0  OutDataTypeStr=uint8
  output1 : Outport
  output2 : Outport  Port=2
  output3 : Outport  Port=3
  output4 : Outport  Port=4
  output5 : Outport  Port=5
  output6 : Outport  Port=6
  output7 : Outport  Port=7
  output8 : Outport  Port=8
  wires:
  ACC_TextInfoForDriver/1 -> ACC_TextInfoForDriver_sat/1
  ACC_TextInfoForDriver_sat/1 -> ACC_TextInfoForDriver_st/1
  ACC_TextInfoForDriver_O/1 -> ACC_TextInfoForDriver_st/2
  ACC_TextInfoForDriver_st/1 -> ACC_TextInfoForDriver_D/1
  ACC_TextInfoForDriver_F/1 -> ACC_TextInfoForDriver_D/2
  ACC_TextInfoForDriver_D/1 -> ACC_TextInfoForDriverRon/1
  ACC_TextInfoForDriverRon/1 -> ACC_TextInfoForDriver_S/1
  ACC_TextInfoForDriver_S/1 -> ACC_TextInfoForDriver_1sat/1
  ACC_TextInfoForDriver_1sat/1 -> ACC_TextInfoForDriver_Convert/1
  ACC_TextInfoForDriver_Convert/1 -> ACC_TextInfoForDriver_L/1
  ACC_TextInfoForDriver_L/1 -> ACC_TextInfoForDriver_D1/1, ACC_TextInfoForDriver_And/1
  ACC_TextInfoForDriveroutput6_C/1 -> ACC_TextInfoForDriver_D1/2
  ACC_TextInfoForDriver_D1/1 -> ACC_TextInfoForDriverCOV/1
  ACC_TextInfoForDriverCOV/1 -> output6/1
  ACC_TextInfoForDriver_And_C/1 -> ACC_TextInfoForDriver_And/2
  ACC_TextInfoForDriver_And/1 -> ACC_TextInfoForDriverBitCov/1
  ACC_TextInfoForDriverBitCov/1 -> output7/1
  Constant1/1 -> output1/1
  Constant2/1 -> output2/1
  Constant3/1 -> output3/1
  Constant4/1 -> output4/1
  Constant5/1 -> output5/1
  Constant8/1 -> output8/1

== system VCU_CS75_12_30_test/长安CS75底盘程序，20ms一次/Output/Subsystem/28A/APA_28A/APA_CheckSum ==
  APA_CheckSum : Inport
  APA_CheckSumRon : Rounding  Operator=round
  APA_CheckSum_1sat : Saturate  UpperLimit=255  LowerLimit=0
  APA_CheckSum_Convert : DataTypeConversion  OutDataTypeStr=uint8
  APA_CheckSum_Convert1 : DataTypeConversion  OutDataTypeStr=uint32
  APA_CheckSum_D : Product  Inputs=*/
  APA_CheckSum_F : Constant  OutDataTypeStr=single
  APA_CheckSum_L : simulink/Logic and Bit Operations/Bitwise Operator  logicop=AND  UseBitMask=on  BitMask=255  BitMaskRealWorld=Stored Integer
  APA_CheckSum_O : Constant  Value=0  OutDataTypeStr=single
  APA_CheckSum_S : ArithShift
  APA_CheckSum_sat : Saturate  UpperLimit=255  LowerLimit=0
  APA_CheckSum_st : Sum  Inputs=+-
  Constant{1..7} (7 alike) : Constant  Value=0  OutDataTypeStr=uint8
  output1 : Outport
  output2 : Outport  Port=2
  output3 : Outport  Port=3
  output4 : Outport  Port=4
  output5 : Outport  Port=5
  output6 : Outport  Port=6
  output7 : Outport  Port=7
  output8 : Outport  Port=8
  wires:
  Constant7/1 -> output7/1
  Constant6/1 -> output6/1
  Constant5/1 -> output5/1
  Constant4/1 -> output4/1
  Constant3/1 -> output3/1
  Constant2/1 -> output2/1
  Constant1/1 -> output1/1
  APA_CheckSum_Convert/1 -> output8/1
  APA_CheckSum_L/1 -> APA_CheckSum_Convert/1
  APA_CheckSum_Convert1/1 -> APA_CheckSum_L/1
  APA_CheckSum_1sat/1 -> APA_CheckSum_Convert1/1
  APA_CheckSum_S/1 -> APA_CheckSum_1sat/1
  APA_CheckSumRon/1 -> APA_CheckSum_S/1
  APA_CheckSum_D/1 -> APA_CheckSumRon/1
  APA_CheckSum_F/1 -> APA_CheckSum_D/2
  APA_CheckSum_st/1 -> APA_CheckSum_D/1
  APA_CheckSum_O/1 -> APA_CheckSum_st/2
  APA_CheckSum_sat/1 -> APA_CheckSum_st/1
  APA_CheckSum/1 -> APA_CheckSum_sat/1

== system VCU_CS75_12_30_test/长安CS75底盘程序，20ms一次/Output/Subsystem/28A/APA_28A/APA_EPSAngleReq ==
  APA_EPSAngleReq : Inport
  APA_EPSAngleReqABS : Abs
  APA_EPSAngleReqBitCov : DataTypeConversion  OutDataTypeStr=uint32
  APA_EPSAngleReqBitCov1 : DataTypeConversion  OutDataTypeStr=uint8
  APA_EPSAngleReqCOV : DataTypeConversion  OutDataTypeStr=uint8
  APA_EPSAngleReqCOV1 : DataTypeConversion  OutDataTypeStr=uint8
  APA_EPSAngleReqCS : ArithShift  BitShiftNumber=-16
  APA_EPSAngleReqConS : Constant  OutDataTypeStr=single
  APA_EPSAngleReqCosR : Constant  Value=0  OutDataTypeStr=uint8
  APA_EPSAngleReqROP : RelationalOperator  Operator=<  OutDataTypeStr=boolean
  APA_EPSAngleReqRon : Rounding  Operator=round
  APA_EPSAngleReqSW : Switch  Criteria=u2 ~= 0
  APA_EPSAngleReq_1sat : Saturate  UpperLimit=1048560  LowerLimit=0
  APA_EPSAngleReq_And : simulink/Logic and Bit Operations/Bitwise Operator  logicop=AND  UseBitMask=off  NumInputPorts=2  BitMask=bin2dec('11011001')  BitMaskRealWorld=Stored Integer
  APA_EPSAngleReq_And1 : simulink/Logic and Bit Operations/Bitwise Operator  logicop=AND  UseBitMask=off  NumInputPorts=2  BitMask=bin2dec('11011001')  BitMaskRealWorld=Stored Integer
  APA_EPSAngleReq_And1_C : Constant  Value=255  OutDataTypeStr=uint32
  APA_EPSAngleReq_And_C : Constant  Value=65535
  APA_EPSAngleReq_Convert : DataTypeConversion  OutDataTypeStr=uint32
  APA_EPSAngleReq_D : Product  Inputs=*/
  APA_EPSAngleReq_D1 : Product  Inputs=*/
  APA_EPSAngleReq_D2 : Product  Inputs=*/
  APA_EPSAngleReq_F : Constant  Value=0.1  OutDataTypeStr=single
  APA_EPSAngleReq_L : simulink/Logic and Bit Operations/Bitwise Operator  logicop=AND  UseBitMask=on  BitMask=1048560  BitMaskRealWorld=Stored Integer
  APA_EPSAngleReq_O : Constant  Value=0  OutDataTypeStr=single
  APA_EPSAngleReq_S : ArithShift  BitShiftNumber=-4
  APA_EPSAngleReq_sat : Saturate  UpperLimit=3276.7  LowerLimit=-3276.8
  APA_EPSAngleReq_st : Sum  Inputs=+-
  APA_EPSAngleReqoutput2_C : Constant  Value=65536
  APA_EPSAngleReqoutput3_C : Constant  Value=256
  APA_EPSAngleReqsubcon : Sum  Inputs=+-
  Constant{1,5..8} (5 alike) : Constant  Value=0  OutDataTypeStr=uint8
  output1 : Outport
  output2 : Outport  Port=2
  output3 : Outport  Port=3
  output4 : Outport  Port=4
  output5 : Outport  Port=5
  output6 : Outport  Port=6
  output7 : Outport  Port=7
  output8 : Outport  Port=8
  wires:
  Constant8/1 -> output8/1
  Constant7/1 -> output7/1
  Constant6/1 -> output6/1
  Constant5/1 -> output5/1
  Constant1/1 -> output1/1
  APA_EPSAngleReqBitCov1/1 -> output4/1
  APA_EPSAngleReq_And1/1 -> APA_EPSAngleReqBitCov1/1
  APA_EPSAngleReq_And1_C/1 -> APA_EPSAngleReq_And1/2
  APA_EPSAngleReqCOV1/1 -> output3/1
  APA_EPSAngleReq_D2/1 -> APA_EPSAngleReqCOV1/1
  APA_EPSAngleReqoutput3_C/1 -> APA_EPSAngleReq_D2/2
  APA_EPSAngleReq_And/1 -> APA_EPSAngleReq_D2/1
  APA_EPSAngleReqBitCov/1 -> APA_EPSAngleReq_And/2
  APA_EPSAngleReq_And_C/1 -> APA_EPSAngleReqBitCov/1
  APA_EPSAngleReqCOV/1 -> output2/1
  APA_EPSAngleReq_D1/1 -> APA_EPSAngleReqCOV/1
  APA_EPSAngleReqoutput2_C/1 -> APA_EPSAngleReq_D1/2
  APA_EPSAngleReq_L/1 -> APA_EPSAngleReq_And1/1, APA_EPSAngleReq_And/1, APA_EPSAngleReq_D1/1
  APA_EPSAngleReq_Convert/1 -> APA_EPSAngleReq_L/1
  APA_EPSAngleReq_1sat/1 -> APA_EPSAngleReq_Convert/1
  APA_EPSAngleReq_S/1 -> APA_EPSAngleReq_1sat/1
  APA_EPSAngleReqSW/1 -> APA_EPSAngleReq_S/1
  APA_EPSAngleReqROP/1 -> APA_EPSAngleReqSW/2
  APA_EPSAngleReqsubcon/1 -> APA_EPSAngleReqSW/1
  APA_EPSAngleReqABS/1 -> APA_EPSAngleReqsubcon/2
  APA_EPSAngleReqCS/1 -> APA_EPSAngleReqsubcon/1
  APA_EPSAngleReqConS/1 -> APA_EPSAngleReqCS/1
  APA_EPSAngleReqCosR/1 -> APA_EPSAngleReqROP/2
  APA_EPSAngleReqRon/1 -> APA_EPSAngleReqSW/3, APA_EPSAngleReqABS/1, APA_EPSAngleReqROP/1
  APA_EPSAngleReq_D/1 -> APA_EPSAngleReqRon/1
  APA_EPSAngleReq_F/1 -> APA_EPSAngleReq_D/2
  APA_EPSAngleReq_st/1 -> APA_EPSAngleReq_D/1
  APA_EPSAngleReq_O/1 -> APA_EPSAngleReq_st/2
  APA_EPSAngleReq_sat/1 -> APA_EPSAngleReq_st/1
  APA_EPSAngleReq/1 -> APA_EPSAngleReq_sat/1

== system VCU_CS75_12_30_test/长安CS75底盘程序，20ms一次/Output/Subsystem/28A/APA_28A/APA_IncreasePressureReq ==
  APA_IncreasePressureReq : Inport
  APA_IncreasePressureReqRon : Rounding  Operator=round
  APA_IncreasePressureReq_1sat : Saturate  UpperLimit=128  LowerLimit=0
  APA_IncreasePressureReq_Convert : DataTypeConversion  OutDataTypeStr=uint8
  APA_IncreasePressureReq_Convert1 : DataTypeConversion  OutDataTypeStr=uint32
  APA_IncreasePressureReq_D : Product  Inputs=*/
  APA_IncreasePressureReq_F : Constant  OutDataTypeStr=single
  APA_IncreasePressureReq_L : simulink/Logic and Bit Operations/Bitwise Operator  logicop=AND  UseBitMask=on  BitMask=128  BitMaskRealWorld=Stored Integer
  APA_IncreasePressureReq_O : Constant  Value=0  OutDataTypeStr=single
  APA_IncreasePressureReq_S : ArithShift  BitShiftNumber=-7
  APA_IncreasePressureReq_sat : Saturate  UpperLimit=0  LowerLimit=0
  APA_IncreasePressureReq_st : Sum  Inputs=+-
  Constant{1,3..8} (7 alike) : Constant  Value=0  OutDataTypeStr=uint8
  output1 : Outport
  output2 : Outport  Port=2
  output3 : Outport  Port=3
  output4 : Outport  Port=4
  output5 : Outport  Port=5
  output6 : Outport  Port=6
  output7 : Outport  Port=7
  output8 : Outport  Port=8
  wires:
  Constant8/1 -> output8/1
  Constant7/1 -> output7/1
  Constant6/1 -> output6/1
  Constant5/1 -> output5/1
  Constant4/1 -> output4/1
  Constant3/1 -> output3/1
  Constant1/1 -> output1/1
  APA_IncreasePressureReq_Convert/1 -> output2/1
  APA_IncreasePressureReq_L/1 -> APA_IncreasePressureReq_Convert/1
  APA_IncreasePressureReq_Convert1/1 -> APA_IncreasePressureReq_L/1
  APA_IncreasePressureReq_1sat/1 -> APA_IncreasePressureReq_Convert1/1
  APA_IncreasePressureReq_S/1 -> APA_IncreasePressureReq_1sat/1
  APA_IncreasePressureReqRon/1 -> APA_IncreasePressureReq_S/1
  APA_IncreasePressureReq_D/1 -> APA_IncreasePressureReqRon/1
  APA_IncreasePressureReq_F/1 -> APA_IncreasePressureReq_D/2
  APA_IncreasePressureReq_st/1 -> APA_IncreasePressureReq_D/1
  APA_IncreasePressureReq_O/1 -> APA_IncreasePressureReq_st/2
  APA_IncreasePressureReq_sat/1 -> APA_IncreasePressureReq_st/1
  APA_IncreasePressureReq/1 -> APA_IncreasePressureReq_sat/1

== system VCU_CS75_12_30_test/长安CS75底盘程序，20ms一次/Output/Subsystem/28A/APA_28A/APA_Indication ==
  APA_Indication : Inport
  APA_IndicationRon : Rounding  Operator=round
  APA_Indication_1sat : Saturate  UpperLimit=56  LowerLimit=0
  APA_Indication_Convert : DataTypeConversion  OutDataTypeStr=uint8
  APA_Indication_Convert1 : DataTypeConversion  OutDataTypeStr=uint32
  APA_Indication_D : Product  Inputs=*/
  APA_Indication_F : Constant  OutDataTypeStr=single
  APA_Indication_L : simulink/Logic and Bit Operations/Bitwise Operator  logicop=AND  UseBitMask=on  BitMask=56  BitMaskRealWorld=Stored Integer
  APA_Indication_O : Constant  Value=0  OutDataTypeStr=single
  APA_Indication_S : ArithShift  BitShiftNumber=-3
  APA_Indication_sat : Saturate  UpperLimit=7  LowerLimit=0
  APA_Indication_st : Sum  Inputs=+-
  Constant{2..8} (7 alike) : Constant  Value=0  OutDataTypeStr=uint8
  output1 : Outport
  output2 : Outport  Port=2
  output3 : Outport  Port=3
  output4 : Outport  Port=4
  output5 : Outport  Port=5
  output6 : Outport  Port=6
  output7 : Outport  Port=7
  output8 : Outport  Port=8
  wires:
  Constant8/1 -> output8/1
  Constant7/1 -> output7/1
  Constant6/1 -> output6/1
  Constant5/1 -> output5/1
  Constant4/1 -> output4/1
  Constant3/1 -> output3/1
  Constant2/1 -> output2/1
  APA_Indication_Convert/1 -> output1/1
  APA_Indication_L/1 -> APA_Indication_Convert/1
  APA_Indication_Convert1/1 -> APA_Indication_L/1
  APA_Indication_1sat/1 -> APA_Indication_Convert1/1
  APA_Indication_S/1 -> APA_Indication_1sat/1
  APA_IndicationRon/1 -> APA_Indication_S/1
  APA_Indication_D/1 -> APA_IndicationRon/1
  APA_Indication_F/1 -> APA_Indication_D/2
  APA_Indication_st/1 -> APA_Indication_D/1
  APA_Indication_O/1 -> APA_Indication_st/2
  APA_Indication_sat/1 -> APA_Indication_st/1
  APA_Indication/1 -> APA_Indication_sat/1

== system VCU_CS75_12_30_test/长安CS75底盘程序，20ms一次/Output/Subsystem/28A/APA_28A/APA_OnOff ==
  APA_OnOff : Inport
  APA_OnOffRon : Rounding  Operator=round
  APA_OnOff_1sat : Saturate  UpperLimit=64  LowerLimit=0
  APA_OnOff_Convert : DataTypeConversion  OutDataTypeStr=uint8
  APA_OnOff_Convert1 : DataTypeConversion  OutDataTypeStr=uint32
  APA_OnOff_D : Product  Inputs=*/
  APA_OnOff_F : Constant  OutDataTypeStr=single
  APA_OnOff_L : simulink/Logic and Bit Operations/Bitwise Operator  logicop=AND  UseBitMask=on  BitMask=64  BitMaskRealWorld=Stored Integer
  APA_OnOff_O : Constant  Value=0  OutDataTypeStr=single
  APA_OnOff_S : ArithShift  BitShiftNumber=-6
  APA_OnOff_sat : Saturate  UpperLimit=0  LowerLimit=0
  APA_OnOff_st : Sum  Inputs=+-
  Constant{2..8} (7 alike) : Constant  Value=0  OutDataTypeStr=uint8
  output1 : Outport
  output2 : Outport  Port=2
  output3 : Outport  Port=3
  output4 : Outport  Port=4
  output5 : Outport  Port=5
  output6 : Outport  Port=6
  output7 : Outport  Port=7
  output8 : Outport  Port=8
  wires:
  Constant8/1 -> output8/1
  Constant7/1 -> output7/1
  Constant6/1 -> output6/1
  Constant5/1 -> output5/1
  Constant4/1 -> output4/1
  Constant3/1 -> output3/1
  Constant2/1 -> output2/1
  APA_OnOff_Convert/1 -> output1/1
  APA_OnOff_L/1 -> APA_OnOff_Convert/1
  APA_OnOff_Convert1/1 -> APA_OnOff_L/1
  APA_OnOff_1sat/1 -> APA_OnOff_Convert1/1
  APA_OnOff_S/1 -> APA_OnOff_1sat/1
  APA_OnOffRon/1 -> APA_OnOff_S/1
  APA_OnOff_D/1 -> APA_OnOffRon/1
  APA_OnOff_F/1 -> APA_OnOff_D/2
  APA_OnOff_st/1 -> APA_OnOff_D/1
  APA_OnOff_O/1 -> APA_OnOff_st/2
  APA_OnOff_sat/1 -> APA_OnOff_st/1
  APA_OnOff/1 -> APA_OnOff_sat/1

== system VCU_CS75_12_30_test/长安CS75底盘程序，20ms一次/Output/Subsystem/28A/APA_28A/APA_RollingCounter ==
  APA_RollingCounter : Inport
  APA_RollingCounterRon : Rounding  Operator=round
  APA_RollingCounter_1sat : Saturate  UpperLimit=15  LowerLimit=0
  APA_RollingCounter_Convert : DataTypeConversion  OutDataTypeStr=uint8
  APA_RollingCounter_Convert1 : DataTypeConversion  OutDataTypeStr=uint32
  APA_RollingCounter_D : Product  Inputs=*/
  APA_RollingCounter_F : Constant  OutDataTypeStr=single
  APA_RollingCounter_L : simulink/Logic and Bit Operations/Bitwise Operator  logicop=AND  UseBitMask=on  BitMask=15  BitMaskRealWorld=Stored Integer
  APA_RollingCounter_O : Constant  Value=0  OutDataTypeStr=single
  APA_RollingCounter_S : ArithShift
  APA_RollingCounter_sat : Saturate  UpperLimit=15  LowerLimit=0
  APA_RollingCounter_st : Sum  Inputs=+-
  Constant{1..6,8} (7 alike) : Constant  Value=0  OutDataTypeStr=uint8
  output1 : Outport
  output2 : Outport  Port=2
  output3 : Outport  Port=3
  output4 : Outport  Port=4
  output5 : Outport  Port=5
  output6 : Outport  Port=6
  output7 : Outport  Port=7
  output8 : Outport  Port=8
  wires:
  Constant8/1 -> output8/1
  Constant6/1 -> output6/1
  Constant5/1 -> output5/1
  Constant4/1 -> output4/1
  Constant3/1 -> output3/1
  Constant2/1 -> output2/1
  Constant1/1 -> output1/1
  APA_RollingCounter_Convert/1 -> output7/1
  APA_RollingCounter_L/1 -> APA_RollingCounter_Convert/1
  APA_RollingCounter_Convert1/1 -> APA_RollingCounter_L/1
  APA_RollingCounter_1sat/1 -> APA_RollingCounter_Convert1/1
  APA_RollingCounter_S/1 -> APA_RollingCounter_1sat/1
  APA_RollingCounterRon/1 -> APA_RollingCounter_S/1
  APA_RollingCounter_D/1 -> APA_RollingCounterRon/1
  APA_RollingCounter_F/1 -> APA_RollingCounter_D/2
  APA_RollingCounter_st/1 -> APA_RollingCounter_D/1
  APA_RollingCounter_O/1 -> APA_RollingCounter_st/2
  APA_RollingCounter_sat/1 -> APA_RollingCounter_st/1
  APA_RollingCounter/1 -> APA_RollingCounter_sat/1

== system VCU_CS75_12_30_test/长安CS75底盘程序，20ms一次/Output/Subsystem/28A/APA_28A/APA_SteeringAngleReqProtection ==
  APA_SteeringAngleReqProtection : Inport
  APA_SteeringAngleReqProtectionRon : Rounding  Operator=round
  APA_SteeringAngleReqProtection_1sat : Saturate  UpperLimit=3  LowerLimit=0
  APA_SteeringAngleReqProtection_Convert : DataTypeConversion  OutDataTypeStr=uint8
  APA_SteeringAngleReqProtection_Convert1 : DataTypeConversion  OutDataTypeStr=uint32
  APA_SteeringAngleReqProtection_D : Product  Inputs=*/
  APA_SteeringAngleReqProtection_F : Constant  OutDataTypeStr=single
  APA_SteeringAngleReqProtection_L : simulink/Logic and Bit Operations/Bitwise Operator  logicop=AND  UseBitMask=on  BitMask=3  BitMaskRealWorld=Stored Integer
  APA_SteeringAngleReqProtection_O : Constant  Value=0  OutDataTypeStr=single
  APA_SteeringAngleReqProtection_S : ArithShift
  APA_SteeringAngleReqProtection_sat : Saturate  UpperLimit=3  LowerLimit=0
  APA_SteeringAngleReqProtection_st : Sum  Inputs=+-
  Constant{1..4,6..8} (7 alike) : Constant  Value=0  OutDataTypeStr=uint8
  output1 : Outport
  output2 : Outport  Port=2
  output3 : Outport  Port=3
  output4 : Outport  Port=4
  output5 : Outport  Port=5
  output6 : Outport  Port=6
  output7 : Outport  Port=7
  output8 : Outport  Port=8
  wires:
  Constant8/1 -> output8/1
  Constant7/1 -> output7/1
  Constant6/1 -> output6/1
  Constant4/1 -> output4/1
  Constant3/1 -> output3/1
  Constant2/1 -> output2/1
  Constant1/1 -> output1/1
  APA_SteeringAngleReqProtection_Convert/1 -> output5/1
  APA_SteeringAngleReqProtection_L/1 -> APA_SteeringAngleReqProtection_Convert/1
  APA_SteeringAngleReqProtection_Convert1/1 -> APA_SteeringAngleReqProtection_L/1
  APA_SteeringAngleReqProtection_1sat/1 -> APA_SteeringAngleReqProtection_Convert1/1
  APA_SteeringAngleReqProtection_S/1 -> APA_SteeringAngleReqProtection_1sat/1
  APA_SteeringAngleReqProtectionRon/1 -> APA_SteeringAngleReqProtection_S/1
  APA_SteeringAngleReqProtection_D/1 -> APA_SteeringAngleReqProtectionRon/1
  APA_SteeringAngleReqProtection_F/1 -> APA_SteeringAngleReqProtection_D/2
  APA_SteeringAngleReqProtection_st/1 -> APA_SteeringAngleReqProtection_D/1
  APA_SteeringAngleReqProtection_O/1 -> APA_SteeringAngleReqProtection_st/2
  APA_SteeringAngleReqProtection_sat/1 -> APA_SteeringAngleReqProtection_st/1
  APA_SteeringAngleReqProtection/1 -> APA_SteeringAngleReqProtection_sat/1

== system VCU_CS75_12_30_test/长安CS75底盘程序，20ms一次/Output/Subsystem/28D/LAS_28D/CRC ==
  CRC : Inport
  CRCRon : Rounding  Operator=round
  CRC_1sat : Saturate  UpperLimit=255  LowerLimit=0
  CRC_Convert : DataTypeConversion  OutDataTypeStr=uint8
  CRC_Convert1 : DataTypeConversion  OutDataTypeStr=uint32
  CRC_D : Product  Inputs=*/
  CRC_F : Constant  OutDataTypeStr=single
  CRC_L : simulink/Logic and Bit Operations/Bitwise Operator  logicop=AND  UseBitMask=on  BitMask=255  BitMaskRealWorld=Stored Integer
  CRC_O : Constant  Value=0  OutDataTypeStr=single
  CRC_S : ArithShift
  CRC_sat : Saturate  UpperLimit=0  LowerLimit=0
  CRC_st : Sum  Inputs=+-
  Constant{1..7} (7 alike) : Constant  Value=0  OutDataTypeStr=uint8
  output1 : Outport
  output2 : Outport  Port=2
  output3 : Outport  Port=3
  output4 : Outport  Port=4
  output5 : Outport  Port=5
  output6 : Outport  Port=6
  output7 : Outport  Port=7
  output8 : Outport  Port=8
  wires:
  CRC/1 -> CRC_sat/1
  CRC_sat/1 -> CRC_st/1
  CRC_O/1 -> CRC_st/2
  CRC_st/1 -> CRC_D/1
  CRC_F/1 -> CRC_D/2
  CRC_D/1 -> CRCRon/1
  CRCRon/1 -> CRC_S/1
  CRC_S/1 -> CRC_1sat/1
  CRC_1sat/1 -> CRC_Convert1/1
  CRC_Convert1/1 -> CRC_L/1
  CRC_L/1 -> CRC_Convert/1
  CRC_Convert/1 -> output8/1
  Constant1/1 -> output1/1
  Constant2/1 -> output2/1
  Constant3/1 -> output3/1
  Constant4/1 -> output4/1
  Constant5/1 -> output5/1
  Constant6/1 -> output6/1
  Constant7/1 -> output7/1
